simulink model "flc"  (Simulink 8.8)
settings: Solver=ode45  StartTime=0.0  StopTime=3  RelTol=1e-3  EnableMultiTasking=on
undefined symbols (not defined in the file or in its folder): sigbuilder_block
libraries: fuzblock x1
CloseFcn:
  | rtwprivate ssgencode ModelCloseRequest sima_elegxou
settings Model: Creator=Athina  LastModifiedBy=user  ModifiedComment=Athina -- Sun Aug 13 09:36:28 2017 -- Version 1.21
settings Model: ModifiedHistory=|
  | Athina -- Sun Aug 13 09:36:28 2017 -- Version 1.21
  | 
  | 
  | Athina -- Sat Aug 12 23:41:28 2017 -- Version 1.20
settings SolverCC: ZeroCrossAlgorithm=Adaptive
settings DataIOCC: ExternalInput=[t, y_3]  LimitDataPoints=off
settings OptimizationCC: ExpressionDepthLimit=2147483647
settings DebuggingCC: IgnoredZcDiagnostic=none  StateNameClashWarn=none
settings HardwareCC: TargetHWDeviceType=32-bit Generic  ProdEqTarget=off

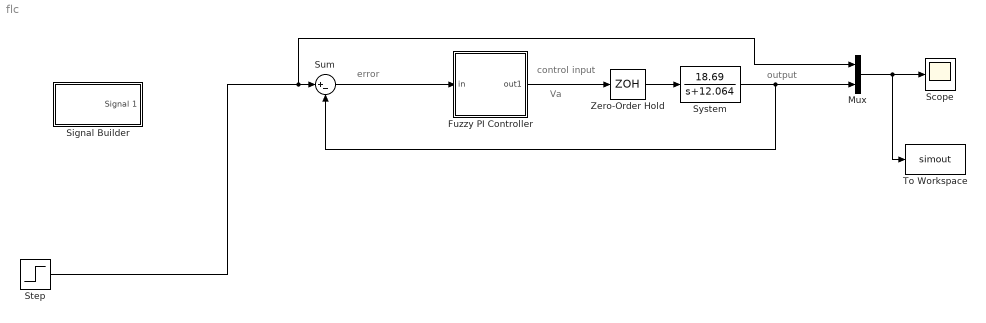
== system flc ==
  note: error
  note: control input
  note: Va
  note: output
  Fuzzy PI Controller : Subsystem
  Mux : Mux  Inputs=2
  Scope : Scope
  Signal Builder : Subsystem  Tag=STV Subsys  LoadFcn=sigbuilder_block('load');  StartFcn=sigbuilder_block('start');  StopFcn=sigbuilder_block('stop');  ClipboardFcn=sigbuilder_block('clipboard');  mask(Sigbuilder block){tuvar=[0:10]}
      mask help: Simulink:masks:SigbuilderBlock_MD
      mask init:
      | if ~strcmp(get_param(bdroot(gcbh),'SimulationStatus'),'stopped') tuvar = sigbuilder_block('maskInit'); end
      settings: CopyFcn=sigbuilder_block('copy');  DeleteFcn=sigbuilder_block('delete');  ModelCloseFcn=sigbuilder_block('modelClose');  PreSaveFcn=sigbuilder_block('preSave');  PauseFcn=sigbuilder_block('pause');  ContinueFcn=sigbuilder_block('continue');  NameChangeFcn=sigbuilder_block('namechange');  OpenFcn=sigbuilder_block('open',[438 189.75 549 389.25 ]);  CloseFcn=sigbuilder_block('close');
      mask Display: plot(0, 0, 100, 100,[2, 2, 32, 32, 2], [68, 8, 8, 68, 68],[32, 2], [38, 38], [32, 19, 2],[53, 60, 44], [32, 17, 17, 2],[16, 16, 31, 31]);txt = getActiveGroup(gcbh);text(2, 100, txt,'verticalAlignment', 'top');
  Step : Step  Time=0  After=150  SampleTime=0
  Sum : Sum  Inputs=|+-
  System : TransferFcn  Numerator=[18.69]  Denominator=[1 12.064]
  To Workspace : ToWorkspace  VariableName=simout  SampleTime=-1
  Zero-Order Hold : ZeroOrderHold
  wires:
  Zero-Order Hold/1 -> System/1
  Mux/1 -> To Workspace/1, Scope/1
  System/1 -> Mux/2, Sum/2
  Sum/1 -> Fuzzy PI Controller/1(in)
  Fuzzy PI Controller/1(out1) -> Zero-Order Hold/1
  Step/1 -> Mux/1, Sum/1

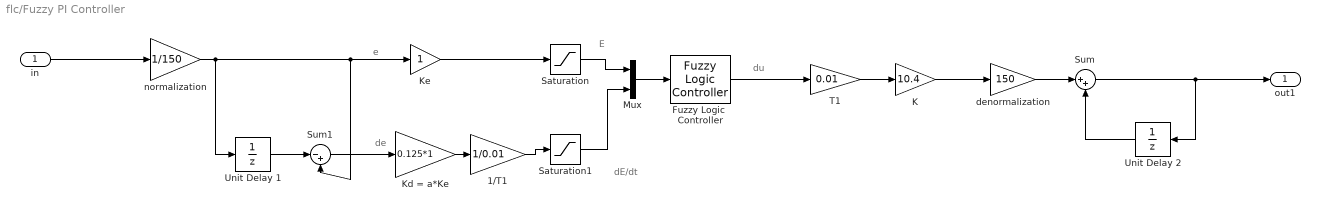
== system flc/Fuzzy PI Controller ==
  note: dE/dt
  note: E
  note: e
  note: de
  note: du
  in : Inport
  1/T1 : Gain  Gain=1/0.01
  Fuzzy Logic  Controller : fuzblock/Fuzzy Logic  Controller  fis='dc.fis'
  K : Gain  Gain=10.4
  Kd = a*Ke : Gain  Gain=0.125*1
  Ke : Gain
  Mux : Mux  Inputs=2
  Saturation : Saturate  UpperLimit=1  LowerLimit=-1
  Saturation1 : Saturate  UpperLimit=1  LowerLimit=-1
  Sum : Sum  Inputs=|++
  Sum1 : Sum  Inputs=|-+
  T1 : Gain  Gain=0.01
  Unit Delay 1 : UnitDelay  SampleTime=-1
  Unit Delay 2 : UnitDelay  SampleTime=-1
  denormalization : Gain  Gain=150
  normalization : Gain  Gain=1/150
  out1 : Outport
  wires:
  normalization/1 -> Unit Delay 1/1, Ke/1, Sum1/2
  Ke/1 -> Saturation/1
  T1/1 -> K/1
  K/1 -> denormalization/1
  denormalization/1 -> Sum/1
  Unit Delay 2/1 -> Sum/2
  Sum/1 -> Unit Delay 2/1, out1/1
  Saturation1/1 -> Mux/2
  1/T1/1 -> Saturation1/1
  Kd = a*Ke/1 -> 1/T1/1
  Unit Delay 1/1 -> Sum1/1
  Sum1/1 -> Kd = a*Ke/1
  in/1 -> normalization/1
  Saturation/1 -> Mux/1
  Mux/1 -> Fuzzy Logic  Controller/1
  Fuzzy Logic  Controller/1 -> T1/1

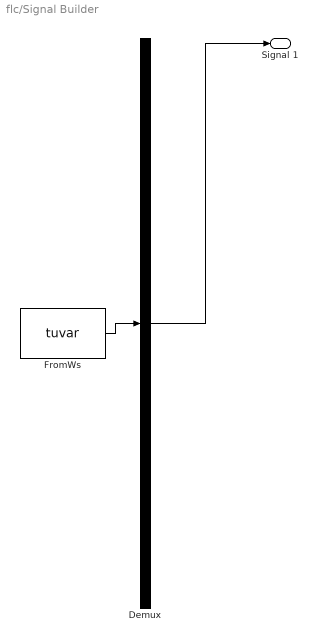
== system flc/Signal Builder ==
  Demux : Demux  Tag=STV Demux  Outputs=1
  FromWs : FromWorkspace  Tag=STV FromWs  VariableName=tuvar  SampleTime=0  SigBuilderData=DataTag0  VnvData=DataTag1
      SigBuilderData=|
      | common.afterFinalStr = 'Extrapolate'
      | common.sampleTime = 0
      | dataSet.timeRange = [0 30]
      | dataSet.name = 'Group 1'
      | sbobj.Groups.Name = 'Group 1'
      | sbobj.Groups.Signals.Name = 'Signal 1'
      | sbobj.Groups.Signals.XData = [0 10 10 20 20 30]
      | sbobj.Groups.Signals.YData = [150 150 100 100 150 150]
      | sbobj.Groups.TimeRange = [0 30]
  Signal 1 : Outport  Tag=STV Outport
  wires:
  Demux/1 -> Signal 1/1
  FromWs/1 -> Demux/1
